simulink model "prob_6_model"  (R2016a)
settings: Solver=FixedStepDiscrete  StartTime=0.0  StopTime=10.0  RelTol=1e-3
values from neighbouring files (symbols this model uses):
  a1 = 1    [Prob_6_mat.mat]
  a2 = 2    [Prob_6_mat.mat]
  a3 = 3    [Prob_6_mat.mat]
  a4 = 4    [Prob_6_mat.mat]
  a5 = 5    [Prob_6_mat.mat]
settings Model: Creator=Admin  LastModifiedBy=Admin

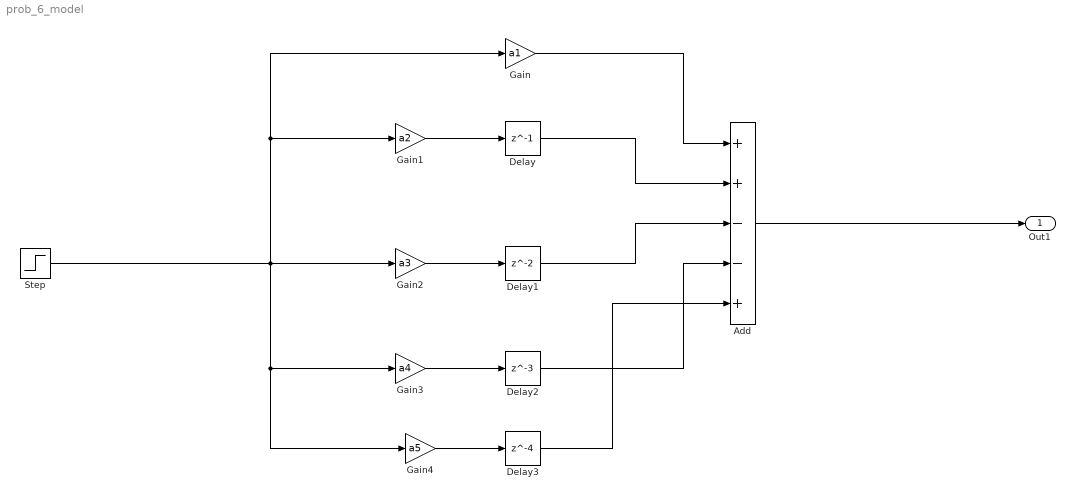
== system prob_6_model ==
  Add : Sum  Inputs=++--+
  Delay : Delay  DelayLength=1
  Delay1 : Delay
  Delay2 : Delay  DelayLength=3
  Delay3 : Delay  DelayLength=4
  Gain : Gain  Gain=a1
  Gain1 : Gain  Gain=a2
  Gain2 : Gain  Gain=a3
  Gain3 : Gain  Gain=a4
  Gain4 : Gain  Gain=a5
  Step : Step  SampleTime=0
  Out1 : Outport
  wires:
  Add/1 -> Out1/1
  Gain1/1 -> Delay/1
  Delay2/1 -> Add/4
  Gain4/1 -> Delay3/1
  Delay1/1 -> Add/3
  Step/1 -> Gain1/1, Gain/1, Gain2/1, Gain3/1, Gain4/1
  Delay/1 -> Add/2
  Gain3/1 -> Delay2/1
  Gain2/1 -> Delay1/1
  Delay3/1 -> Add/5
  Gain/1 -> Add/1
